simulink model "Lab6Task"  (R2016b)
settings: Solver=VariableStepAuto  StartTime=0.0  StopTime=1  RelTol=1e-3
libraries: dsparch4 x1
settings Model: Creator=mahbu  LastModifiedBy=mahbu

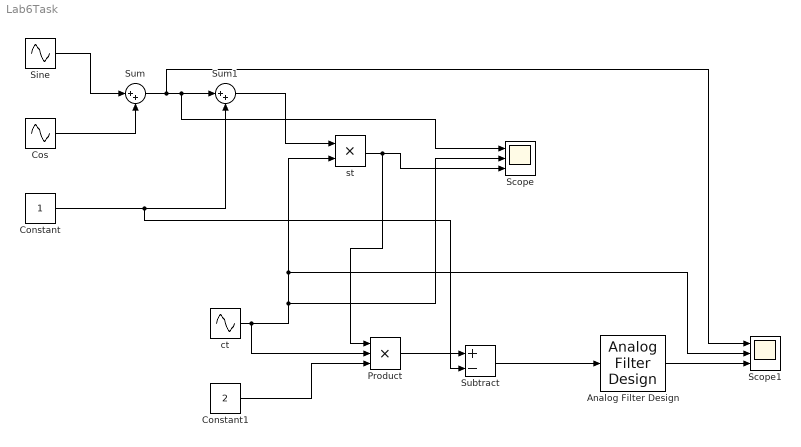
== system Lab6Task ==
  Analog Filter Design : dsparch4/Analog Filter Design  method=Butterworth  filttype=Lowpass  N=8  Wlo=2*pi*8  Whi=80  Rp=2  Rs=40
  Constant : Constant
  Constant1 : Constant  Value=2
  Cos : Sin  Amplitude=3  Frequency=2*pi*6  Phase=pi/2  SampleTime=0
  Product : Product  Inputs=3
  Scope : Scope  NumInputPorts=3
  Scope1 : Scope  NumInputPorts=3
  Sine : Sin  Amplitude=2  Frequency=2*pi*4  SampleTime=0
  Subtract : Sum  Inputs=+-
  Sum : Sum  Inputs=|++
  Sum1 : Sum  Inputs=|++
  "ct " : Sin  Frequency=2*pi*50  Phase=pi/2  SampleTime=0
  "st " : Product
  wires:
  Cos/1 -> Sum/2
  Sine/1 -> Sum/1
  Sum/1 -> Scope1/1, Scope/1, Sum1/1
  Constant/1 -> Subtract/2, Sum1/2
  "ct "/1 -> Product/2, Scope/2, Scope1/2, "st "/2
  Sum1/1 -> "st "/1
  "st "/1 -> Product/1, Scope/3
  Constant1/1 -> Product/3
  Product/1 -> Subtract/1
  Subtract/1 -> Analog Filter Design/1
  Analog Filter Design/1 -> Scope1/3
